simulink model "MSD_Model_Real"  (R2024b)
settings: Solver=VariableStepAuto  StartTime=0.0  StopTime=10.0  RelTol=1e-3
values from neighbouring files (symbols this model uses):
  C = sysD.C    [MSDScript.m]
  delta_x_hat0 = x0 - x_bar    [MSDScript.m]
  G = sysD.A    [MSDScript.m]
  H = sysD.B    [MSDScript.m]
  Kd = place(G, H, desiredPoles)    [MSDScript.m]
  Ld = place(G', C', exp(10*desiredPoles_cont*Ts))'    [MSDScript.m]
  student_ID = 11908203    [MSDScript.m]    (also in MSD_Dynamics_org.m = 0)
  Ts = 0.001    [MSDScript.m]
  u_bar = 5    [MSDScript.m]    (also in createObserverController.m = u_bar(:))
  x0 = [1; 0] + x_bar    [MSDScript.m]
  x_bar = x_bar(:)    [MSDScript.m]    (also in createObserverController.m)
  y_bar = x_bar(1)    [MSDScript.m]    (also in createObserverController.m = Cd * x_bar)
settings Model: Creator=froessil  LastModifiedBy=froessil

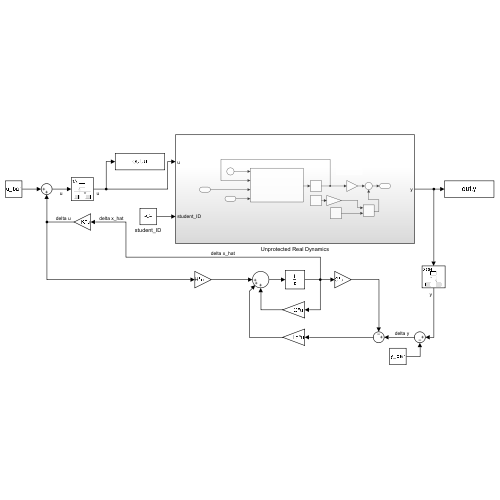
[thumbnail: Simulink's stored preview of the top-level diagram]
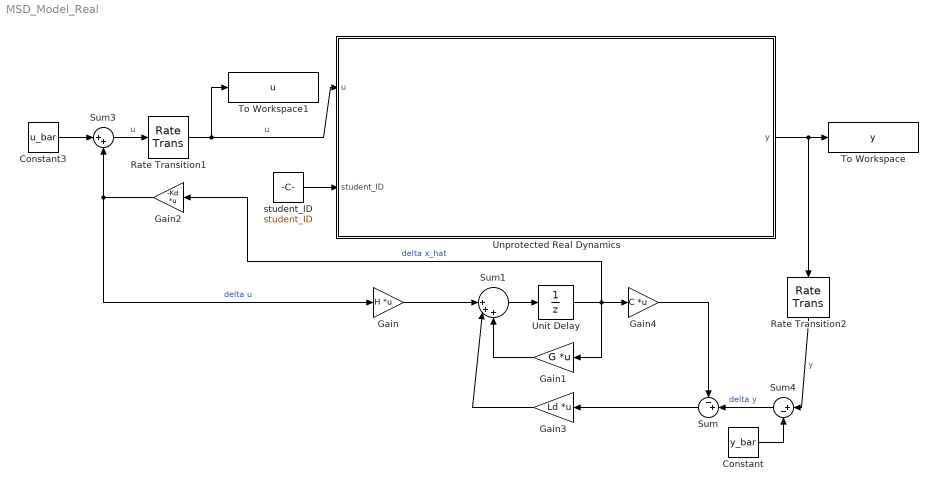
== system MSD_Model_Real ==
  Constant : Constant  Value=y_bar
  Constant3 : Constant  Value=u_bar
  Gain : Gain  Gain=H  Multiplication=Matrix(K*u)
  Gain1 : Gain  Gain=G  Multiplication=Matrix(K*u)
  Gain2 : Gain  Gain=-Kd  Multiplication=Matrix(K*u)
  Gain3 : Gain  Gain=Ld  Multiplication=Matrix(K*u)
  Gain4 : Gain  Gain=C  Multiplication=Matrix(K*u)
  Rate Transition1 : RateTransition  InitialCondition=-Kd*(x0-x_bar)+u_bar  OutPortSampleTime=0
  Rate Transition2 : RateTransition  InitialCondition=x0(1)  OutPortSampleTime=Ts
  Sum : Sum  Inputs=-+|
  Sum1 : Sum  Inputs=||+++
  Sum3 : Sum  Inputs=|++
  Sum4 : Sum  Inputs=|+-
  To Workspace : ToWorkspace  VariableName=y  SaveFormat=Timeseries  SampleTime=-1
  To Workspace1 : ToWorkspace  VariableName=u  SaveFormat=Timeseries  SampleTime=-1
  Unit Delay : UnitDelay  InitialCondition=delta_x_hat0  SampleTime=-1  HasFrameUpgradeWarning=on
  Unprotected Real Dynamics : Subsystem
  student_ID : Constant  Value=student_ID
  wires:
  Gain2/1 -> Sum3/2, Gain/1  "delta u"
  Constant3/1 -> Sum3/1
  Sum3/1 -> Rate Transition1/1  "u"
  Gain/1 -> Sum1/1
  Gain3/1 -> Sum1/2
  Unit Delay/1 -> Gain2/1, Gain1/1, Gain4/1  "delta x_hat"
  Unprotected Real Dynamics/1(y) -> To Workspace/1, Rate Transition2/1
  Sum/1 -> Gain3/1
  Gain4/1 -> Sum/1
  Sum1/1 -> Unit Delay/1
  Rate Transition1/1 -> To Workspace1/1, Unprotected Real Dynamics/1(u)  "u"
  Gain1/1 -> Sum1/3
  Sum4/1 -> Sum/2  "delta y"
  Constant/1 -> Sum4/2
  Rate Transition2/1 -> Sum4/1  "y"
  student_ID/1 -> Unprotected Real Dynamics/2(student_ID)

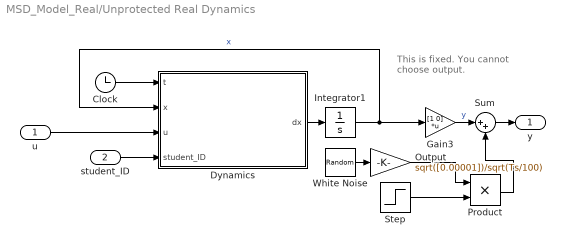
== system MSD_Model_Real/Unprotected Real Dynamics ==
  note: This is fixed. You cannot choose output.
  u : Inport
  student_ID : Inport  Port=2
  Clock : Clock
  "Dynamics " : MATLAB Function  TreatAsAtomicUnit=on
  Gain3 : Gain  Gain=[1 0]  Multiplication=Matrix(K*u)
  Integrator1 : Integrator  InitialCondition=x0
  Output : Gain  Gain=sqrt([0.00001])/sqrt(Ts/100)  SaturateOnIntegerOverflow=on  OutDataTypeStr=Inherit: Same as input  ParamDataTypeStr=Inherit: Same as input
  Product : Product
  Step : Step  Time=0  After=.1  SampleTime=0
  Sum : Sum  Inputs=|++
  White Noise : RandomNumber  DisableCoverage=on  Seed=student_ID  SampleTime=Ts/100
  y : Outport
  wires:
  Step/1 -> Product/2
  student_ID/1 -> "Dynamics "/4(student_ID)
  u/1 -> "Dynamics "/3(u)
  Gain3/1 -> Sum/1  "y"
  Clock/1 -> "Dynamics "/1(t)
  Sum/1 -> y/1
  White Noise/1 -> Output/1
  Integrator1/1 -> "Dynamics "/2(x), Gain3/1  "x"
  Output/1 -> Product/1
  Product/1 -> Sum/2
  "Dynamics "/1(dx) -> Integrator1/1

== matlab function MSD_Model_Real/Unprotected Real Dynamics/Dynamics  ==
  data: t input; x input; u input; student_ID input; dx output
function dx = MSD_Dynamics_Testing(t, x, u, student_ID)
dx = zeros(2,1);
dx = MSD_Dynamics(t, x, u, student_ID);
